simulink model "Pipe_p_to_p_test"  (R2014b)
settings: Solver=ode45  StartTime=0.0  StopTime=10.0  RelTol=1e-3
libraries: DAEMOT_Lib x3
settings Model: Creator=pangbor2  LastModifiedBy=koeln2

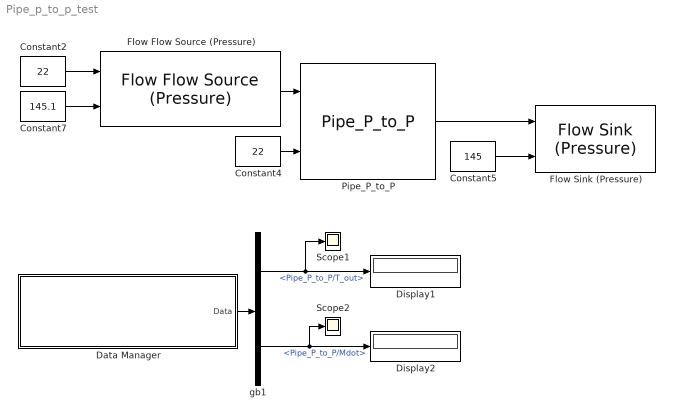
== system Pipe_p_to_p_test ==
  Constant2 : Constant  Value=22
  Constant4 : Constant  Value=22
  Constant5 : Constant  Value=145
  Constant7 : Constant  Value=145.1
  Data Manager : Subsystem  AncestorBlock=DAEMOT_Lib/Support Functions/Data Manager  mask{null=0}
      mask init:
      | set_param(gcb, 'LinkStatus', 'inactive')    % disable the library link
      settings: OpenFcn=data_manager
      mask Display: str ='Pipe_P_to_P/T_out\nPipe_P_to_P/Mdot'; fprintf(str)
  Display1 : Display
  Display2 : Display
  Flow Flow Source (Pressure) : DAEMOT_Lib/Components/Flow Flow Source (Pressure)  M_ext=on  M=0  T_ext=on  T=0  P_ext=on  P=0
  Flow Sink (Pressure) : DAEMOT_Lib/Components/Flow Sink (Pressure)  M_ext=on  M=0  T_ext=on  T=0  P_ext=on  P=0
  Pipe_P_to_P : DAEMOT_Lib/Components/Pipe_P_to_P  fld=Water  T_init=22  Tamb_init=22  f=0.05  KL=0  H=0  D=13*1e-3  L=0.2  t=0.0015  E=0.01*1e-3  v=0.4  e_rough=0.01*1e-3
  Scope1 : Scope
  Scope2 : Scope
  gb1 : BusSelector  OutputSignals=Pipe_P_to_P/T_out,Pipe_P_to_P/Mdot
  wires:
  Constant7/1 -> Flow Flow Source (Pressure)/2
  Constant2/1 -> Flow Flow Source (Pressure)/1
  Flow Flow Source (Pressure)/1 -> Pipe_P_to_P/1
  Constant5/1 -> Flow Sink (Pressure)/2
  Pipe_P_to_P/1 -> Flow Sink (Pressure)/1
  Constant4/1 -> Pipe_P_to_P/2
  Data Manager/1(Data) -> gb1/1
  gb1/1 -> Scope1/1, Display1/1  "<Pipe_P_to_P/T_out>"
  gb1/2 -> Scope2/1, Display2/1  "<Pipe_P_to_P/Mdot>"

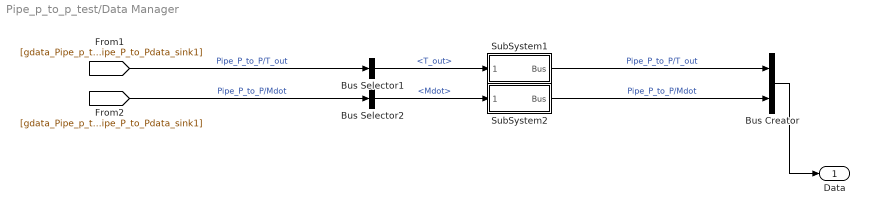
== system Pipe_p_to_p_test/Data Manager ==
  Bus Creator : BusCreator  Inputs=2
  Bus Selector1 : BusSelector  OutputSignals=T_out
  Bus Selector2 : BusSelector  OutputSignals=Mdot
  SubSystem1 : Subsystem
  SubSystem2 : Subsystem
  Data : Outport
  wires:
  Bus Creator/1 -> Data/1
  [gdata_Pipe_p_to_p_testPipe_P_to_Pdata_sink1] -> Bus Selector1/1  "Pipe_P_to_P/T_out"
  Bus Selector1/1 -> SubSystem1/1(Rename)  "<T_out>"
  SubSystem1/1(Bus) -> Bus Creator/1  "Pipe_P_to_P/T_out"
  [gdata_Pipe_p_to_p_testPipe_P_to_Pdata_sink1] -> Bus Selector2/1  "Pipe_P_to_P/Mdot"
  Bus Selector2/1 -> SubSystem2/1(Rename)  "<Mdot>"
  SubSystem2/1(Bus) -> Bus Creator/2  "Pipe_P_to_P/Mdot"

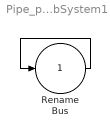
== system Pipe_p_to_p_test/Data Manager/SubSystem1 ==
  Rename : Inport
  Bus : Outport
  wires:
  Rename/1 -> Bus/1

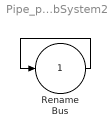
== system Pipe_p_to_p_test/Data Manager/SubSystem2 ==
  Rename : Inport
  Bus : Outport
  wires:
  Rename/1 -> Bus/1
